simulink model "opt_plan"  (R2024a)
settings: Solver=FixedStepAuto  StartTime=0.0  StopTime=100  FixedStep=ts  RelTol=1e-3
values from neighbouring files (symbols this model uses):
  A = [A1; A2; A3; A4; A5; A6]    [setup.m]
  B = [0, 0 ... (first row only)    [setup.m]
  C = [0, 0, 1, 0, 0, 0 ... (first row only)    [setup.m]
  D = [0 0 ... (first row only)    [setup.m]
  Ig = 10*(m*l^2)/3    (= 6)    [setup.m]
  m = 5    [setup.m]
  ni_r = 1    [setup.m]
  ni_x = 1    [setup.m]
  ni_y = 6    [setup.m]
  ts = 0.02    [setup.m]
  u_eq = [m*g; 0]    [setup.m]
  w = [1,      1 ... (first row only)    [setup.m]
  z_eq = z_init    [setup.m]
  z_init = [0;0;0;0;0;0]    [setup.m]
libraries: slpidlib x3
settings Model: Creator=enead  LastModifiedBy=enead

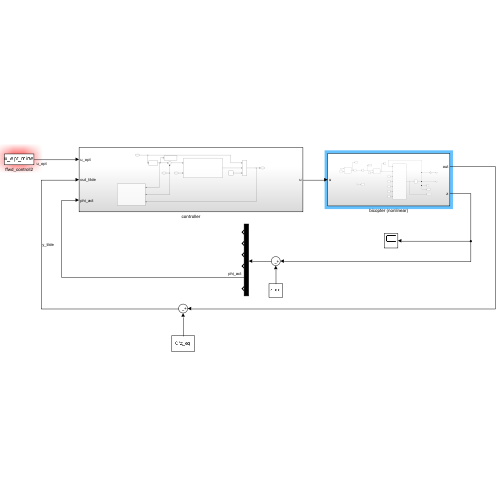
[thumbnail: Simulink's stored preview of the top-level diagram]
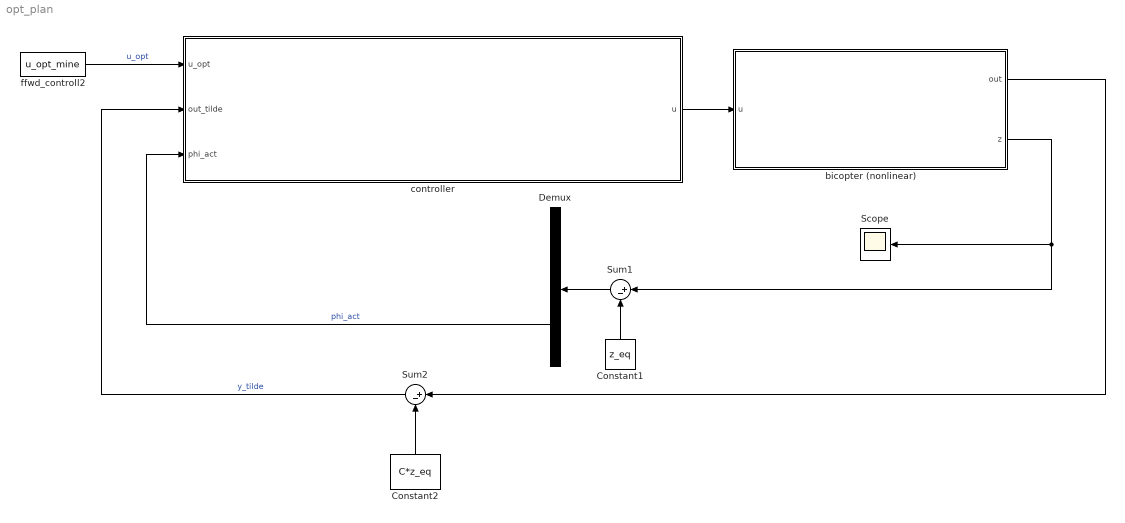
== system opt_plan ==
  Constant1 : Constant  Value=z_eq
  Constant2 : Constant  Value=C*z_eq
  Demux : Demux  Outputs=6
  Scope : Scope
  Sum1 : Sum  Inputs=|+-
  Sum2 : Sum  Inputs=|+-
  bicopter (nonlinear) : Subsystem
  controller : Subsystem
  ffwd_controll2 : FromWorkspace  VariableName=u_opt_mine  SampleTime=ts  OutputAfterFinalValue=Holding final value
  wires:
  Constant1/1 -> Sum1/2
  Sum1/1 -> Demux/1
  bicopter (nonlinear)/1(out) -> Sum2/1
  Constant2/1 -> Sum2/2
  bicopter (nonlinear)/2(z) -> Scope/1, Sum1/1
  Demux/5 -> controller/3(phi_act)  "phi_act"
  Sum2/1 -> controller/2(out_tilde)  "y_tilde"
  controller/1(u) -> bicopter (nonlinear)/1(u)
  ffwd_controll2/1 -> controller/1(u_opt)  "u_opt"

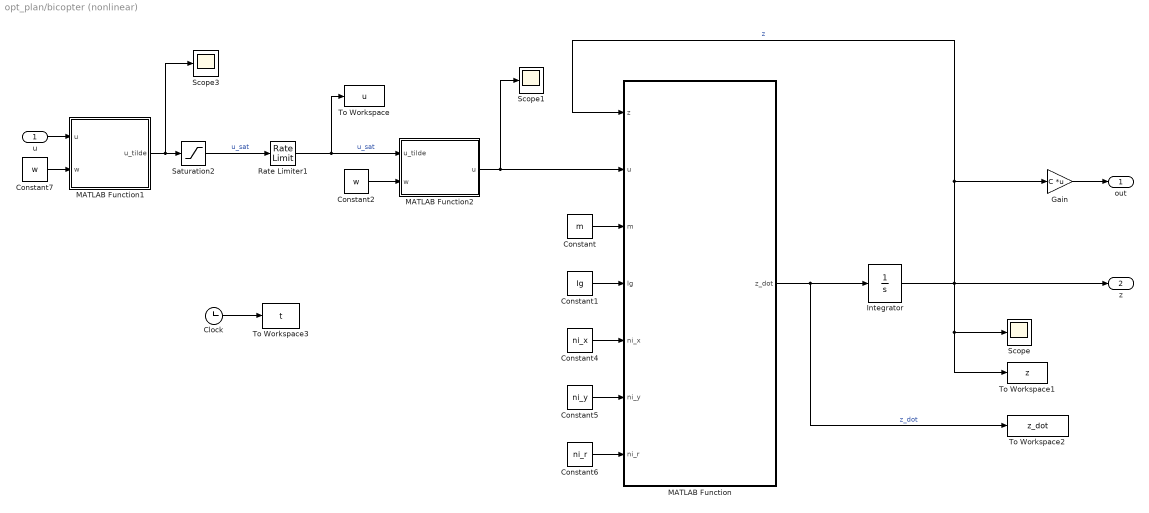
== system opt_plan/bicopter (nonlinear) ==
  u : Inport
  Clock : Clock
  Constant : Constant  Value=m
  Constant1 : Constant  Value=Ig
  Constant2 : Constant  Value=w
  Constant4 : Constant  Value=ni_x
  Constant5 : Constant  Value=ni_y  VectorParams1D=off
  Constant6 : Constant  Value=ni_r
  Constant7 : Constant  Value=w
  Gain : Gain  Gain=C  Multiplication=Matrix(K*u)
  Integrator : Integrator  InitialCondition=z_init
  MATLAB Function : MATLAB Function  TreatAsAtomicUnit=on
  MATLAB Function1 : MATLAB Function  TreatAsAtomicUnit=on
  MATLAB Function2 : MATLAB Function  TreatAsAtomicUnit=on
  Rate Limiter1 : RateLimiter  RisingSlewLimit=10  FallingSlewLimit=-10  SampleTimeMode=inherited
  Saturation2 : Saturate  UpperLimit=100  LowerLimit=0
  Scope : Scope
  Scope1 : Scope
  Scope3 : Scope
  To Workspace : ToWorkspace  VariableName=u  SaveFormat=Timeseries  SampleTime=-1
  To Workspace1 : ToWorkspace  VariableName=z  SaveFormat=Timeseries  SampleTime=-1
  To Workspace2 : ToWorkspace  VariableName=z_dot  SaveFormat=Timeseries  SampleTime=-1
  To Workspace3 : ToWorkspace  VariableName=t  SaveFormat=Timeseries  SampleTime=-1
  out : Outport
  z : Outport  Port=2
  wires:
  Constant1/1 -> MATLAB Function/4(Ig)
  Integrator/1 -> Gain/1, MATLAB Function/1(z), z/1, To Workspace1/1, Scope/1  "z"
  Constant/1 -> MATLAB Function/3(m)
  MATLAB Function/1(z_dot) -> To Workspace2/1, Integrator/1  "z_dot"
  u/1 -> MATLAB Function1/1(u)
  Constant4/1 -> MATLAB Function/5(ni_x)
  Constant5/1 -> MATLAB Function/6(ni_y)
  Constant6/1 -> MATLAB Function/7(ni_r)
  MATLAB Function1/1(u_tilde) -> Saturation2/1, Scope3/1
  MATLAB Function2/1(u) -> MATLAB Function/2(u), Scope1/1
  Constant2/1 -> MATLAB Function2/2(w)
  Constant7/1 -> MATLAB Function1/2(w)
  Clock/1 -> To Workspace3/1
  Gain/1 -> out/1
  Rate Limiter1/1 -> To Workspace/1, MATLAB Function2/1(u_tilde)  "u_sat"
  Saturation2/1 -> Rate Limiter1/1  "u_sat"

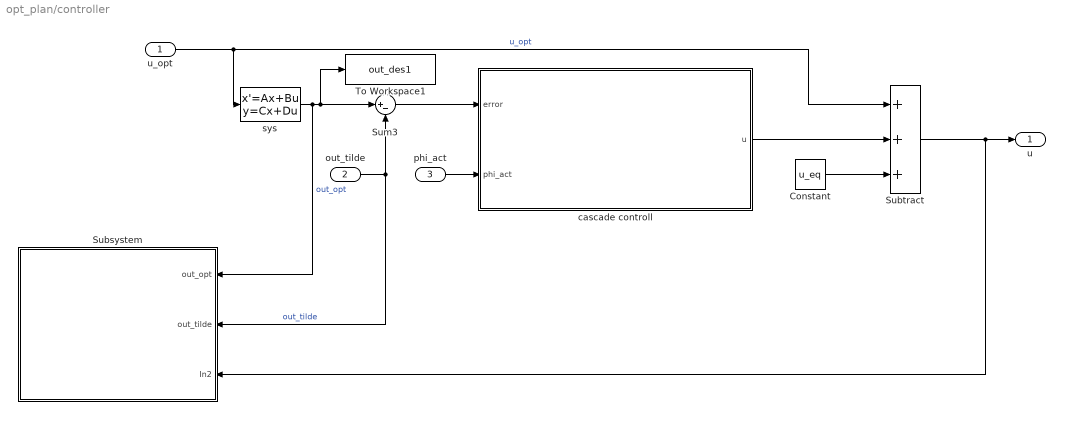
== system opt_plan/controller ==
  u_opt : Inport
  out_tilde : Inport  Port=2
  phi_act : Inport  Port=3
  Constant : Constant  Value=u_eq
  Subsystem : Subsystem
  Subtract : Sum  Inputs=+++
  Sum3 : Sum  Inputs=|+-
  To Workspace1 : ToWorkspace  VariableName=out_des1  SaveFormat=Timeseries  SampleTime=-1
  cascade controll : Subsystem
  sys : StateSpace  A=A  B=B  C=C  D=D  InitialCondition=0
  u : Outport
  wires:
  cascade controll/1(u) -> Subtract/2
  Sum3/1 -> cascade controll/1(error)
  Constant/1 -> Subtract/3
  phi_act/1 -> cascade controll/2(phi_act)
  u_opt/1 -> sys/1, Subtract/1  "u_opt"
  Subtract/1 -> Subsystem/3(In2), u/1
  sys/1 -> Sum3/1, To Workspace1/1, Subsystem/1(out_opt)  "out_opt"
  out_tilde/1 -> Subsystem/2(out_tilde), Sum3/2  "out_tilde"

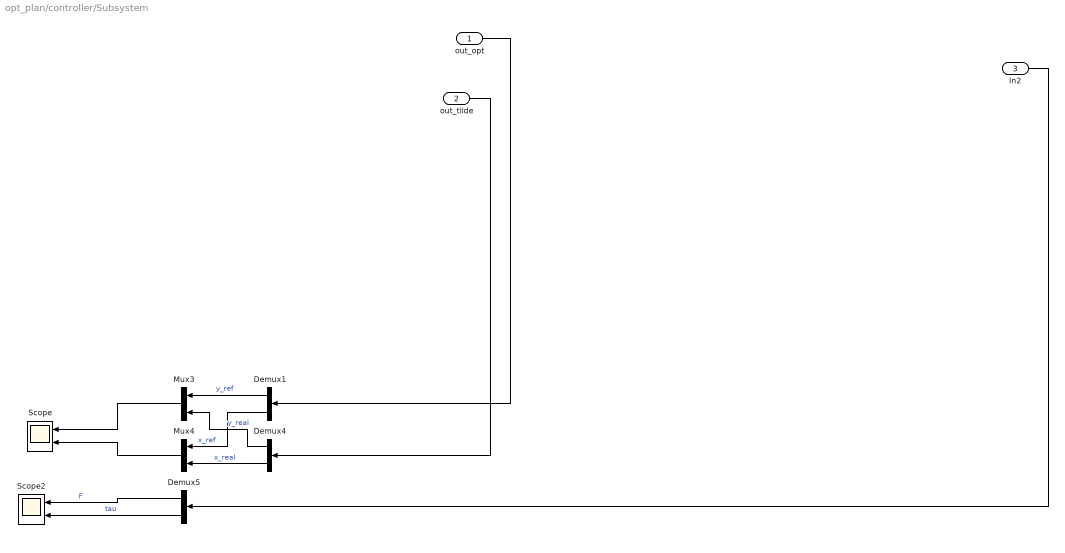
== system opt_plan/controller/Subsystem ==
  out_opt : Inport
  out_tilde : Inport  Port=2
  In2 : Inport  Port=3
  Demux1 : Demux  Outputs=2
  Demux4 : Demux  Outputs=2
  Demux5 : Demux  Outputs=2
  Mux3 : Mux  Inputs=2
  Mux4 : Mux  Inputs=2
  Scope : Scope  NumInputPorts=2
  Scope2 : Scope  NumInputPorts=2
  wires:
  Demux4/1 -> Mux3/2  "y_real"
  Demux1/1 -> Mux3/1  "y_ref"
  Mux4/1 -> Scope/2
  Demux4/2 -> Mux4/2  "x_real"
  Demux1/2 -> Mux4/1  "x_ref"
  out_opt/1 -> Demux1/1
  Demux5/2 -> Scope2/2  "tau"
  Mux3/1 -> Scope/1
  Demux5/1 -> Scope2/1  "F"
  out_tilde/1 -> Demux4/1
  In2/1 -> Demux5/1

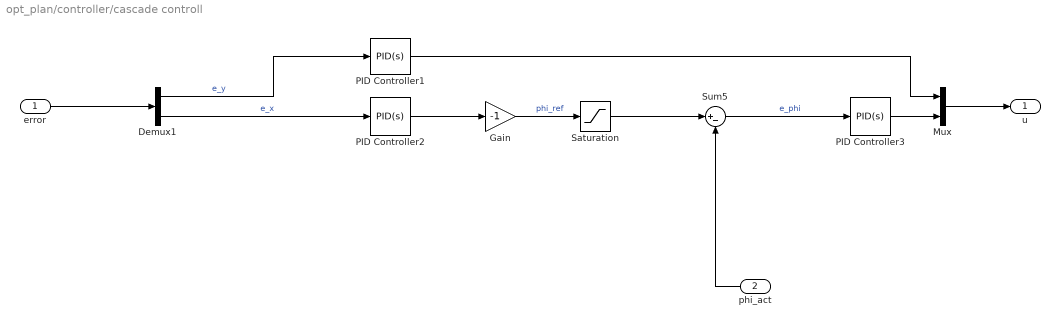
== system opt_plan/controller/cascade controll ==
  error : Inport
  phi_act : Inport  Port=2
  Demux1 : Demux  Outputs=2
  Gain : Gain  Gain=-1
  Mux : Mux  Inputs=2
  PID Controller1 : slpidlib/PID Controller  Controller=PID  Form=Parallel  TimeDomain=Continuous-time  UseExternalTs=off  SampleTime=-1  IntegratorMethod=Forward Euler  FilterMethod=Forward Euler  ControllerParametersSource=internal  P=12  I=0  UseKiTs=off  D=13  UseExternalDerivativeSource=off  N=30  UseFilter=on  TunerSelectOption=Transfer Function Based (PID Tuner App)  InitialConditionSource=internal  InitialConditionForIntegrator=0  InitialConditionForFilter=0  DifferentiatorICPrevScaledInput=0  ExternalReset=none  TrackingMode=off  Kt=1  LimitOutput=off  SatLimitsSource=internal  UpperSaturationLimit=inf  LowerSaturationLimit=-inf  LinearizeAsGain=on  AntiWindupMode=none  Kb=1  LimitIntegrator=off  UpperIntegratorSaturationLimit=inf  LowerIntegratorSaturationLimit=-inf  POutMin=[]  POutMax=[]  IOutMin=[]  IOutMax=[]  DOutMin=[]  DOutMax=[]  NOutMin=[]  NOutMax=[]  SumOutMin=[]  SumOutMax=[]  SaturationOutMin=[]  SaturationOutMax=[]  PParamMin=[]  PParamMax=[]  IParamMin=[]  IParamMax=[]  DParamMin=[]  DParamMax=[]  NParamMin=[]  NParamMax=[]  KbParamMin=[]  KbParamMax=[]  KtParamMin=[]  KtParamMax=[]  KbOutMin=[]  KbOutMax=[]  KtOutMin=[]  KtOutMax=[]  IntegratorOutMin=[]  IntegratorOutMax=[]  FilterOutMin=[]  FilterOutMax=[]  SumI1OutMin=[]  SumI1OutMax=[]  SumI2OutMin=[]  SumI2OutMax=[]  SumI3OutMin=[]  SumI3OutMax=[]  SumI4OutMin=[]  SumI4OutMax=[]  SumDOutMin=[]  SumDOutMax=[]  DifferentiatorOutMin=[]  DifferentiatorOutMax=[]  FilterDiffOutCoefMin=[]  FilterDiffOutCoefMax=[]  ReciprocalOutMin=[]  ReciprocalOutMax=[]  SumDenOutMin=[]  SumDenOutMax=[]  SumNumOutMin=[]  SumNumOutMax=[]  DivideOutMin=[]  DivideOutMax=[]  UdiffTsProdOutMin=[]  UdiffTsProdOutMax=[]  NTsProdOutMin=[]  NTsProdOutMax=[]  UintegralTsProdOutMin=[]  UintegralTsProdOutMax=[]  UngainTsProdOutMin=[]  UngainTsProdOutMax=[]  ClampingZeroOutDataTypeStr=Inherit: Inherit via back propagation  ClampingZeroOutMin=[]  ClampingZeroOutMax=[]  FilterDenConstantOutDataTypeStr=Inherit: Inherit via back propagation  FilterDenConstantOutMin=[]  FilterDenConstantOutMax=[]  PCopyOutDataTypeStr=Inherit: Inherit via back propagation  PCopyOutMin=[]  PCopyOutMax=[]  NCopyOutDataTypeStr=Inherit: Inherit via back propagation  NCopyOutMin=[]  NCopyOutMax=[]  IntegratorContinuousStateAttributes=''  IntegratorStateMustResolveToSignalObject=off  IntegratorRTWStateStorageClass=Auto  FilterContinuousStateAttributes=''  FilterStateMustResolveToSignalObject=off  FilterRTWStateStorageClass=Auto  ParallelPVariant=InternalParameters  IdealPVariant=Disabled  IVariant=InternalParameters  DVariant=InternalParameters  IntegratorVariant=Continuous  SatVariant=Disabled  AWVariant=Passthrough  PCopyVariant=Disabled  TRVariant=Disabled  FdbkBlocksVariant=Forward  IdealPFdbkVariant=Disabled  SatFdbkVariant=Disabled  DerivativeFilterVariant=ContFilter  NVariant=InternalParameters  NCopyVariant=Disabled  FilterICVariant=InternalICsFilter  IntegratorICVariant=InternalICs  ExternalResetVariant=Disabled  TRSumVariant=Passthrough  SumFdbkVariant=Disabled  SumVariant=Sum_PID  TsampFilterVariant=InternalTs  TsampNgainVariant=Passthrough  TsampIntegralVariant=Disabled_SignalSpec  ExternalSaturationOutDataTypeStr=Inherit: Same as second input  DerivativeSourceVariant=ErrorSignal
  PID Controller2 : slpidlib/PID Controller  Controller=PID  Form=Parallel  TimeDomain=Continuous-time  UseExternalTs=off  SampleTime=-1  IntegratorMethod=Forward Euler  FilterMethod=Forward Euler  ControllerParametersSource=internal  P=0.09  I=0  UseKiTs=off  D=0.17  UseExternalDerivativeSource=off  N=14  UseFilter=on  TunerSelectOption=Transfer Function Based (PID Tuner App)  InitialConditionSource=internal  InitialConditionForIntegrator=0  InitialConditionForFilter=0  DifferentiatorICPrevScaledInput=0  ExternalReset=none  TrackingMode=off  Kt=1  LimitOutput=off  SatLimitsSource=internal  UpperSaturationLimit=inf  LowerSaturationLimit=-inf  LinearizeAsGain=on  AntiWindupMode=none  Kb=1  LimitIntegrator=off  UpperIntegratorSaturationLimit=inf  LowerIntegratorSaturationLimit=-inf  POutMin=[]  POutMax=[]  IOutMin=[]  IOutMax=[]  DOutMin=[]  DOutMax=[]  NOutMin=[]  NOutMax=[]  SumOutMin=[]  SumOutMax=[]  SaturationOutMin=[]  SaturationOutMax=[]  PParamMin=[]  PParamMax=[]  IParamMin=[]  IParamMax=[]  DParamMin=[]  DParamMax=[]  NParamMin=[]  NParamMax=[]  KbParamMin=[]  KbParamMax=[]  KtParamMin=[]  KtParamMax=[]  KbOutMin=[]  KbOutMax=[]  KtOutMin=[]  KtOutMax=[]  IntegratorOutMin=[]  IntegratorOutMax=[]  FilterOutMin=[]  FilterOutMax=[]  SumI1OutMin=[]  SumI1OutMax=[]  SumI2OutMin=[]  SumI2OutMax=[]  SumI3OutMin=[]  SumI3OutMax=[]  SumI4OutMin=[]  SumI4OutMax=[]  SumDOutMin=[]  SumDOutMax=[]  DifferentiatorOutMin=[]  DifferentiatorOutMax=[]  FilterDiffOutCoefMin=[]  FilterDiffOutCoefMax=[]  ReciprocalOutMin=[]  ReciprocalOutMax=[]  SumDenOutMin=[]  SumDenOutMax=[]  SumNumOutMin=[]  SumNumOutMax=[]  DivideOutMin=[]  DivideOutMax=[]  UdiffTsProdOutMin=[]  UdiffTsProdOutMax=[]  NTsProdOutMin=[]  NTsProdOutMax=[]  UintegralTsProdOutMin=[]  UintegralTsProdOutMax=[]  UngainTsProdOutMin=[]  UngainTsProdOutMax=[]  ClampingZeroOutDataTypeStr=Inherit: Inherit via back propagation  ClampingZeroOutMin=[]  ClampingZeroOutMax=[]  FilterDenConstantOutDataTypeStr=Inherit: Inherit via back propagation  FilterDenConstantOutMin=[]  FilterDenConstantOutMax=[]  PCopyOutDataTypeStr=Inherit: Inherit via back propagation  PCopyOutMin=[]  PCopyOutMax=[]  NCopyOutDataTypeStr=Inherit: Inherit via back propagation  NCopyOutMin=[]  NCopyOutMax=[]  IntegratorContinuousStateAttributes=''  IntegratorStateMustResolveToSignalObject=off  IntegratorRTWStateStorageClass=Auto  FilterContinuousStateAttributes=''  FilterStateMustResolveToSignalObject=off  FilterRTWStateStorageClass=Auto  ParallelPVariant=InternalParameters  IdealPVariant=Disabled  IVariant=InternalParameters  DVariant=InternalParameters  IntegratorVariant=Continuous  SatVariant=Disabled  AWVariant=Passthrough  PCopyVariant=Disabled  TRVariant=Disabled  FdbkBlocksVariant=Forward  IdealPFdbkVariant=Disabled  SatFdbkVariant=Disabled  DerivativeFilterVariant=ContFilter  NVariant=InternalParameters  NCopyVariant=Disabled  FilterICVariant=InternalICsFilter  IntegratorICVariant=InternalICs  ExternalResetVariant=Disabled  TRSumVariant=Passthrough  SumFdbkVariant=Disabled  SumVariant=Sum_PID  TsampFilterVariant=InternalTs  TsampNgainVariant=Passthrough  TsampIntegralVariant=Disabled_SignalSpec  ExternalSaturationOutDataTypeStr=Inherit: Same as second input  DerivativeSourceVariant=ErrorSignal
  PID Controller3 : slpidlib/PID Controller  Controller=PID  Form=Parallel  TimeDomain=Continuous-time  UseExternalTs=off  SampleTime=-1  IntegratorMethod=Forward Euler  FilterMethod=Forward Euler  ControllerParametersSource=internal  P=5  I=0  UseKiTs=off  D=28  UseExternalDerivativeSource=off  N=10  UseFilter=on  TunerSelectOption=Transfer Function Based (PID Tuner App)  InitialConditionSource=internal  InitialConditionForIntegrator=0  InitialConditionForFilter=0  DifferentiatorICPrevScaledInput=0  ExternalReset=none  TrackingMode=off  Kt=1  LimitOutput=off  SatLimitsSource=internal  UpperSaturationLimit=inf  LowerSaturationLimit=-inf  LinearizeAsGain=on  AntiWindupMode=none  Kb=1  LimitIntegrator=off  UpperIntegratorSaturationLimit=inf  LowerIntegratorSaturationLimit=-inf  POutMin=[]  POutMax=[]  IOutMin=[]  IOutMax=[]  DOutMin=[]  DOutMax=[]  NOutMin=[]  NOutMax=[]  SumOutMin=[]  SumOutMax=[]  SaturationOutMin=[]  SaturationOutMax=[]  PParamMin=[]  PParamMax=[]  IParamMin=[]  IParamMax=[]  DParamMin=[]  DParamMax=[]  NParamMin=[]  NParamMax=[]  KbParamMin=[]  KbParamMax=[]  KtParamMin=[]  KtParamMax=[]  KbOutMin=[]  KbOutMax=[]  KtOutMin=[]  KtOutMax=[]  IntegratorOutMin=[]  IntegratorOutMax=[]  FilterOutMin=[]  FilterOutMax=[]  SumI1OutMin=[]  SumI1OutMax=[]  SumI2OutMin=[]  SumI2OutMax=[]  SumI3OutMin=[]  SumI3OutMax=[]  SumI4OutMin=[]  SumI4OutMax=[]  SumDOutMin=[]  SumDOutMax=[]  DifferentiatorOutMin=[]  DifferentiatorOutMax=[]  FilterDiffOutCoefMin=[]  FilterDiffOutCoefMax=[]  ReciprocalOutMin=[]  ReciprocalOutMax=[]  SumDenOutMin=[]  SumDenOutMax=[]  SumNumOutMin=[]  SumNumOutMax=[]  DivideOutMin=[]  DivideOutMax=[]  UdiffTsProdOutMin=[]  UdiffTsProdOutMax=[]  NTsProdOutMin=[]  NTsProdOutMax=[]  UintegralTsProdOutMin=[]  UintegralTsProdOutMax=[]  UngainTsProdOutMin=[]  UngainTsProdOutMax=[]  ClampingZeroOutDataTypeStr=Inherit: Inherit via back propagation  ClampingZeroOutMin=[]  ClampingZeroOutMax=[]  FilterDenConstantOutDataTypeStr=Inherit: Inherit via back propagation  FilterDenConstantOutMin=[]  FilterDenConstantOutMax=[]  PCopyOutDataTypeStr=Inherit: Inherit via back propagation  PCopyOutMin=[]  PCopyOutMax=[]  NCopyOutDataTypeStr=Inherit: Inherit via back propagation  NCopyOutMin=[]  NCopyOutMax=[]  IntegratorContinuousStateAttributes=''  IntegratorStateMustResolveToSignalObject=off  IntegratorRTWStateStorageClass=Auto  FilterContinuousStateAttributes=''  FilterStateMustResolveToSignalObject=off  FilterRTWStateStorageClass=Auto  ParallelPVariant=InternalParameters  IdealPVariant=Disabled  IVariant=InternalParameters  DVariant=InternalParameters  IntegratorVariant=Continuous  SatVariant=Disabled  AWVariant=Passthrough  PCopyVariant=Disabled  TRVariant=Disabled  FdbkBlocksVariant=Forward  IdealPFdbkVariant=Disabled  SatFdbkVariant=Disabled  DerivativeFilterVariant=ContFilter  NVariant=InternalParameters  NCopyVariant=Disabled  FilterICVariant=InternalICsFilter  IntegratorICVariant=InternalICs  ExternalResetVariant=Disabled  TRSumVariant=Passthrough  SumFdbkVariant=Disabled  SumVariant=Sum_PID  TsampFilterVariant=InternalTs  TsampNgainVariant=Passthrough  TsampIntegralVariant=Disabled_SignalSpec  ExternalSaturationOutDataTypeStr=Inherit: Same as second input  DerivativeSourceVariant=ErrorSignal
  Saturation : Saturate  UpperLimit=2  LowerLimit=-2
  Sum5 : Sum  Inputs=|+-
  u : Outport
  wires:
  Saturation/1 -> Sum5/1
  PID Controller2/1 -> Gain/1
  Demux1/2 -> PID Controller2/1  "e_x"
  PID Controller3/1 -> Mux/2
  Sum5/1 -> PID Controller3/1  "e_phi"
  PID Controller1/1 -> Mux/1
  Demux1/1 -> PID Controller1/1  "e_y"
  Gain/1 -> Saturation/1  "phi_ref"
  phi_act/1 -> Sum5/2
  error/1 -> Demux1/1
  Mux/1 -> u/1

== matlab function opt_plan/bicopter (nonlinear)/MATLAB Function ==
  data: z input; u input; z_dot output; m input; Ig input; ni_x input; ni_y input; ni_r input
function z_dot = drone_nonlinear_evol(z, u, m, Ig, ni_x, ni_y, ni_r)

    g = 9.81;

    x = z(1);
    x_dot = z(2);
    y = z(3);
    y_dot = z(4);
    phi = z(5);
    phi_dot = z(6);

    F = u(1);
    tau = u(2);

    z_dot1 = x_dot;
    z_dot2 = - F/m * sin(phi) - ni_x*x_dot*sin(phi)/m;
    z_dot3 = y_dot;
    z_dot4 = F/m * cos(phi) - g  - ni_y*y_dot*cos(phi)/m;
    z_dot5 = phi_dot;
    z_dot6 = tau/Ig - ni_r*phi_dot/Ig;

    z_dot = [z_dot1; z_dot2; z_dot3; z_dot4; z_dot5; z_dot6];

== matlab function opt_plan/bicopter (nonlinear)/MATLAB Function1 ==
  data: u input; u_tilde output; w input
function u_tilde = tilding(u, w)

    u_tilde = w\u;

== matlab function opt_plan/bicopter (nonlinear)/MATLAB Function2 ==
  data: u_tilde input; u output; w input
function u = detilding(u_tilde, w)

    u = w*u_tilde;
